simulink model "helicopter_sim"  (R2024b)
settings: Solver=ode4  StartTime=0.0  StopTime=30  FixedStep=ST  RelTol=1e-3
StopFcn:
  | % main rotor flapping restraint
  | if over_flap
  |     warning('MyModel:flapping', '<strong> main rotor blade flapping exceeded limits </strong>');
  | end
  | % tail rotor flapping restraint
  | if over_flap_tr
  |     warning('MyModel:flapping_tr', '<strong> tail rotor blade flapping exceeded limits </strong>');
  | end
  | % main rotor load limit
  | if load_mr
  |     warning('MyModel:load_mr', '<strong> main rotor load limit reached </strong>');
  | end
  | % main rotor power limit
  | if power_mr
  |     warning('MyModel:power_mr', '<strong> transmission maximum power rating reached </strong>');
  | end
  | % main rotor blade stall
  | if stall_mr
  |     warning('MyModel:blade_stall', '<strong> main rotor blade stall </strong>');
  | end
  | clear over_flap over_flap_tr load_mr power_mr stall_mr
values from neighbouring files (symbols this model uses):
  a_0 = [ 0 0 0 ]'*pi/180    [parameters.m]    (also in trim.m = [ flap_ss(1) flap_ss(2) flap_ss(3) ]')
  a_hs = 6    [parameters.m]
  a_vs = 6    [parameters.m]
  AKBETA = 0    [parameters.m]
  AKONE = 0    [parameters.m]
  AKONETR = tan(30*(pi/180))    [parameters.m]
  alpha_stall = 15    [parameters.m]
  AOP = 0    [parameters.m]
  AOPTR = 0    [parameters.m]
  AR_hs = 4.5    [parameters.m]
  AR_vs = 1.8    [parameters.m]
  ASLOPE = 6    [parameters.m]
  ASLOPETR = 6    [parameters.m]
  BLADES = 4    [parameters.m]
  BLADESTR = 3    [parameters.m]
  BLCG = 0    [parameters.m]
  BLHS = 0    [parameters.m]
  BLMR = 0    [parameters.m]
  BLRPF = 0    [parameters.m]
  BLTR = -1.8*Ft_m    (= -0.54864)    [parameters.m]
  BLVS = 0    [parameters.m]
  CD_f = [1.774 0.2043 7]    [parameters.m]
  CD_mr = [0.0107 -0.151 1.72]    [parameters.m]
  CD_tr = [ 0.0107 -0.151 1.72 ]    [parameters.m]
  chi_mr = 1    [parameters.m]
  chi_tr = 1    [parameters.m]
  CHORD = 2*Ft_m    (= 0.6096)    [parameters.m]
  CHORDTR = 1*Ft_m    (= 0.3048)    [parameters.m]
  CL_f = [-0.4279 10.33]    [parameters.m]
  CL_max_hs = 1.2    [parameters.m]
  CL_max_vs = 1.2    [parameters.m]
  CLL_f = [0.0696 6.336]    [parameters.m]
  CM_f = [-4.4961 49.522]    [parameters.m]
  CN_f = [0.0396 -21.699]    [parameters.m]
  CY_f = [-0.0359 -16.987]    [parameters.m]
  D = zeros(9,4)    [linearization.m]
  dyn_viscosity = 17.89e-6    (= 1.789e-05)    [parameters.m]
  e_hs = 0.8    [parameters.m]
  e_vs = 0.8    [parameters.m]
  EPSLN = 0.05    [parameters.m]
  euler0 = [ 0 0 0 ]'*pi/180    [parameters.m]    (also in trim.m = [ euler_trim(1)*abs(max_att) euler_trim(2)*abs(max_att) eule)
  fc = [  100*Kn_mps ... (first row only)    [parameters.m]
  GAMMA = 8.1    [parameters.m]
  GAMMATR = 4    [parameters.m]
  href = 0    [parameters.m]
  i_hs = -3*(pi/180)+a0_hs    (= -0.0523598775598)    [parameters.m]
  i_s = 0    [parameters.m]
  i_vs = 0*(pi/180)+a0_vs    (= -0.0872664625997)    [parameters.m]
  Jbeta = 1/3*m_blade*ROTOR^3*(1-EPSLN)^3    (= 3891.86391298)    [parameters.m]
  k_ind = 1    [parameters.m]
  k_ind_tr = 1    [parameters.m]
  kv_tr = 0.8    [parameters.m]
  Lambda_hs = 13*(pi/180)    (= 0.226892802759)    [parameters.m]
  Lambda_vs = 27*(pi/180)    (= 0.471238898038)    [parameters.m]
  lat_cyc_range = [ -15 15 ]    [parameters.m]
  latref = 39.24744998520548    (= 39.2474499852)    [parameters.m]
  lon_cyc_range = [ -15 15 ]    [parameters.m]
  lonref = 9.050782438199448    (= 9.0507824382)    [parameters.m]
  m = 20000*Lb_Kg    (= 9071.84)    [parameters.m]
  m_blade = 0.372*Slug_Kg/Ft_m    (= 17.8114564173)    [parameters.m]
  max_flap_mr = 20*pi/180    (= 0.349065850399)    [parameters.m]
  max_flap_tr = 20*pi/180    (= 0.349065850399)    [parameters.m]
  max_load = 3*m*9.81    (= 266984.2512)    [parameters.m]
  mode = 0    [linearization.m]    (also in parameters.m; trim.m)
  mr_coll_range = [   0 25 ]    [parameters.m]
  OMEGA = 206.9*(pi/30)    (= 21.6665173343)    [parameters.m]
  omega0 = [ 0 0 0 ]'    [parameters.m]
  OMEGATR = 954.93*(pi/30)    (= 100.000035756)    [parameters.m]
  pilot_trim = [ x(1); x(2); x(3); x(4) ]    [trim.m]
  rated_power = 4170*hp_W    (= 3109569)    [parameters.m]
  ROTOR = 30*Ft_m    (= 9.144)    [parameters.m]
  ROTORTR = 6.5*Ft_m    (= 1.9812)    [parameters.m]
  S_hs = 18*(Ft_m^2)    (= 1.67225472)    [parameters.m]
  S_vs = 33*(Ft_m^2)    (= 3.06580032)    [parameters.m]
  ST = 0.001    [parameters.m]
  STACG = 24.4*Ft_m    (= 7.43712)    [parameters.m]
  STAHS = 57.4*Ft_m    (= 17.49552)    [parameters.m]
  STAMR = 23.9*Ft_m    (= 7.28472)    [parameters.m]
  STARPF = 23.9*Ft_m    (= 7.28472)    [parameters.m]
  STATR = 61.4*Ft_m    (= 18.71472)    [parameters.m]
  STAVS = 59.4*Ft_m    (= 18.10512)    [parameters.m]
  THETT = -10*(pi/180)    (= -0.174532925199)    [parameters.m]
  THETTTR = -5*(pi/180)    (= -0.0872664625997)    [parameters.m]
  tr_coll_range = [   0 20 ]    [parameters.m]
  Ttrb = [ 1 0 0; 0 0 1; 0 -1 0]    [parameters.m]
  V0 = eul2rotm(euler0','XYZ')'*[ fc(1) fc(2) fc(3) ]'    [parameters.m]    (also in trim.m)
  wind_rate = [ 0 0 0 ]'    [parameters.m]
  wind_velocity_e = [ 0 0 0 ]'    [parameters.m]
  WLCG = 9.2*Ft_m    (= 2.80416)    [parameters.m]
  WLHS = 7.7*Ft_m    (= 2.34696)    [parameters.m]
  WLMR = 16.7*Ft_m    (= 5.09016)    [parameters.m]
  WLRPF = 12.2*Ft_m    (= 3.71856)    [parameters.m]
  WLTR = 15.2*Ft_m    (= 4.63296)    [parameters.m]
  WLVS = 12.2*Ft_m    (= 3.71856)    [parameters.m]
  Xe_0 = [ 16404 0 -1000 ]'*Ft_m    [parameters.m]
undefined symbols (not defined in the file or in its folder): Earth, rad, s, WGS84
libraries: simulink x4, aerolibanimutils x2, aerolibsim3d x2, sim3dlib x1, aerolibconvert2 x1, shared6dof x1, aerolibtransform2 x1, aerolibatmos2 x1
(part 3 of 3)

== matlab function helicopter_sim/HELICOPTER MODEL/HELICOPTER FORCES AND MOMENTS/MAIN ROTOR/AERODYNAMIC AND INERTIAL FORCES AND MOMENTS ==
  data: chi input; i_s input; m_blade input; Jbeta input; GAMMA input; EPSLN input; AKBETA input; g input; BLADES input; Mrotor output; ASLOPE input; AKONE input; CHORD input; CD input; ROTOR input; A1s input; B1s input; a0 input; a1 input; b1 input; a0dot input; a1dot input; b1dot input; a0ddot input; a1ddot input; b1ddot input; Theta0 input; THETT input; dyn_viscosity input; k_ind input; STACG input; BLCG input; WLCG input; STAH input; BLH input; WLH input; rho input; TAS input; omega_TAS input; Frotor output; omega input; OMEGA input; lambda_i output; lambda output; T output; Q output; alpha_loc output
function [Mrotor,Frotor,lambda_i,lambda,T,Q,alpha_loc]  = fcn(chi,i_s,m_blade,Jbeta,GAMMA,EPSLN,AKBETA,g,BLADES,ASLOPE,AKONE,CHORD,CD,ROTOR,A1s,B1s,...
                                                                    a0,a1,b1,a0dot,a1dot,b1dot,a0ddot,a1ddot,b1ddot,Theta0,THETT,dyn_viscosity,k_ind,...
                                                                    STACG,BLCG,WLCG,STAH,BLH,WLH,rho,TAS,omega_TAS,omega,OMEGA)

%% preliminary calculations
A = pi*ROTOR^2; % area of rotor disc 
sigma = BLADES*CHORD/(pi*ROTOR); % solidity of rotor 
lever_arm_H = [STACG-STAH BLH-BLCG WLCG-WLH]'; % vector from cg to rotor hub
TAS_H = [1 chi 1]'.*(TAS + cross(omega_TAS,lever_arm_H)); % wind speed at rotor
% rotation of airspeed from body to hub-body frame:
uH = TAS_H(1)*cos(i_s)-TAS_H(3)*sin(i_s);
vH = TAS_H(2);
wH = TAS_H(1)*sin(i_s)+TAS_H(3)*cos(i_s);
beta_w = atan2(vH,uH); % sideslip angle 
Mu = sqrt(uH^2+vH^2)/(OMEGA*ROTOR); % advance ratio
p = omega(1); % roll rate
q = omega(2); % pitch rate
r = omega(3); % yaw rate
% rotation of body angular rates from body to hub-body frame:
pH = chi*(p*cos(i_s)+r*sin(i_s));
qH = q;
% rotation of body angular rates from hub-body to hub-wind frame:
pW = pH*cos(beta_w)+qH*sin(beta_w);
qW = -pH*sin(beta_w)+qH*cos(beta_w);
% rotation of feathering angles from hub-body to hub-wind frame:
A1c = A1s*cos(beta_w)-B1s*sin(beta_w);
B1c = A1s*sin(beta_w)+B1s*cos(beta_w);
Mbeta = g*1/2*m_blade*ROTOR^2*(1-EPSLN)^2; % weight moment of the blade around flap hinge (small flapping angle beta and level attitude) 
                                           % (distance from blade c.g. to flap hinge)*(blade weight) [N*m]
                                           % small contribution to the coning angle, can be neglected

%% thrust and inflow calculation

lambda = fzero(@(x) x-wH/(OMEGA*ROTOR)+0.5*(0.5*BLADES*rho*ASLOPE*CHORD*ROTOR*(OMEGA*ROTOR)^2*(1/2*(1-EPSLN^2)*x+Theta0*(1/3+Mu^2/2*(1-EPSLN))+THETT*(1/4+Mu^2/4*(1-EPSLN^2))+...
                    -Mu/2*(1-EPSLN^2)*(B1c-AKONE*b1)-a0*(1/3+Mu^2/2*(1-EPSLN))*AKONE+a1*(Mu/2*EPSLN*(1-EPSLN))-a0dot/OMEGA*(1/3-EPSLN/2)+b1dot/OMEGA*(Mu/4*(1-EPSLN)^2)+...
                    +Mu/4*(1-EPSLN^2)*pW/OMEGA)-BLADES*Mbeta/g*a0ddot)/(rho*A*(OMEGA*ROTOR)^2)/sqrt(Mu^2+x^2), -0.1);
vi = wH-lambda*OMEGA*ROTOR;
lambda_i = -vi/OMEGA/ROTOR;
T =  0.5*BLADES*rho*ASLOPE*CHORD*ROTOR*(OMEGA*ROTOR)^2*(1/2*(1-EPSLN^2)*lambda+Theta0*(1/3+Mu^2/2*(1-EPSLN))+THETT*(1/4+Mu^2/4*(1-EPSLN^2))+...
     -Mu/2*(1-EPSLN^2)*(B1c-AKONE*b1)-a0*(1/3+Mu^2/2*(1-EPSLN))*AKONE+a1*(Mu/2*EPSLN*(1-EPSLN))-a0dot/OMEGA*(1/3-EPSLN/2)+b1dot/OMEGA*(Mu/4*(1-EPSLN)^2)+...
     +Mu/4*(1-EPSLN^2)*pW/OMEGA)-BLADES*Mbeta/g*a0ddot;
CT = T/(rho*A*(OMEGA*ROTOR)^2);
V = sqrt(vi^2+(OMEGA*ROTOR)^2);
Re = rho*CHORD*V/dyn_viscosity; % Reynolds number based on tip speed and rotor chord
alpha_mean = 6*CT/ASLOPE/sigma;
delta = CD(1)+CD(2)*alpha_mean+CD(3)*alpha_mean^2;

%% forces and moments in the hub-wind frame

H_w = BLADES/2*rho*ASLOPE*CHORD*ROTOR*(OMEGA*ROTOR)^2*(delta*Mu/(2*ASLOPE)*(1-EPSLN^2)-1/4*(Theta0-AKONE*a0)*(2*lambda*Mu*(1-EPSLN)+ ...
      -Mu*(1-EPSLN)^2*a0dot/OMEGA-(EPSLN-2/3)*(b1dot/OMEGA-a1)-2/3*a1+2/3*pW/OMEGA)-THETT/4*(Mu*lambda*(1-EPSLN^2)+a0dot/OMEGA*Mu*(EPSLN-2/3)+...
      -2*(EPSLN/3-1/4)*(b1dot/OMEGA-a1)-a1/2+1/2*pW/OMEGA)+1/4*(A1c-AKONE*a1)*(-b1*Mu/4*(1-EPSLN^2)+1/4*Mu*(1-EPSLN)^2*(a1dot/OMEGA+b1)+2/3*a0+...
      +Mu/4*(1-EPSLN^2)*qW/OMEGA)+1/4*(B1c-AKONE*b1)*(3/4*Mu*(1-EPSLN)^2*(b1dot/OMEGA-a1)+(1-EPSLN^2)*(lambda-a1*Mu/4)+(EPSLN-2/3)*a0dot/OMEGA+...
      +3*Mu/4*(1-EPSLN^2)*pW/OMEGA)+1/4*(EPSLN*(1-EPSLN)*(b1dot/OMEGA-a1)*4*lambda-(1-EPSLN^2)*(2*lambda*(b1dot/OMEGA-a1)-a1*lambda)+...
      -(2/3-EPSLN)*(a1*a0dot/OMEGA+a0*(a1dot/OMEGA+b1))-2*a0/3*qW/OMEGA-(2*(1-EPSLN^2)*lambda-4*(1/3-EPSLN/2)*a0dot/OMEGA)*pW/OMEGA+...
      +4*a0dot/OMEGA*(b1dot/OMEGA-a1)*(1/3-EPSLN+EPSLN^2))+Mu/4*(EPSLN*(1-EPSLN)*(a1*(b1dot/OMEGA-a1)+b1*(a1dot/OMEGA+b1))+...
      +1/4*(1-EPSLN)^2*(b1*(a1dot/OMEGA+b1)+a1*(b1dot/OMEGA-a1))-1/2*(1-EPSLN^2)*(a1*(b1dot/OMEGA-a1)+b1*(a1dot/OMEGA+b1)-2*a0^2-b1^2/2-3/2*a1^2)+...
      -a1/4*(1-EPSLN^2)*pW/OMEGA-b1/4*(1-EPSLN^2)*qW/OMEGA));

Y_w = BLADES/2*rho*ASLOPE*CHORD*ROTOR*(OMEGA*ROTOR)^2*(-1/4*(Theta0-AKONE*a0)*(((EPSLN-2/3)*(a1dot/OMEGA+b1)-2/3*b1)+3*a0*(1-EPSLN^2)*Mu+ ...
      -2*b1*(1-EPSLN)*Mu^2-2/3*qW/OMEGA)-THETT/4*(((2/3*EPSLN-1/2)*(a1dot/OMEGA+b1)-b1/2)+2*a0*Mu-b1*(1-EPSLN^2)*Mu^2+ ...
      -1/2*qW/OMEGA)-1/4*(A1c-AKONE*a1)*(((EPSLN-2/3)*a0dot/OMEGA+lambda*(1-EPSLN^2))+Mu*(5/4*a1*(1-EPSLN^2)+1/4*(1-EPSLN)^2*(b1dot/OMEGA-a1))+...
      +Mu/4*(1-EPSLN^2)*pW/OMEGA)-1/4*(B1c-AKONE*b1)*(-2/3*a0+Mu*(7/4*b1*(1-EPSLN^2)+1/4*(1-EPSLN)^2*(a1dot/OMEGA+b1)+...
      +1/4*qW/OMEGA)-Mu^2*(2*a0*(1-EPSLN)))-1/4*(4*(1/3-EPSLN+EPSLN^2)*a0dot/OMEGA*(a1dot/OMEGA+b1)-2*lambda*(1-EPSLN)^2*(a1dot/OMEGA+b1)+...
      +2/3*a0*pW/OMEGA+2*a0*(1/3-EPSLN/2)*(b1dot/OMEGA-a1)-2*b1*(lambda/2*(1-EPSLN^2)-a0dot/OMEGA*(1/3-EPSLN/2))+(4*(1/3-EPSLN/2)*a0dot/OMEGA+...
      -2*(1-EPSLN^2)*lambda)*qW/OMEGA)-Mu/4*(6*a0*lambda*(1-EPSLN)-a1*b1/2*(1-EPSLN^2)-3*(1-EPSLN)^2*a0*a0dot/OMEGA-7/4*(1-EPSLN)^2*a1*(a1dot/OMEGA+b1)+...
      -5/4*b1*(1-EPSLN^2)*pW/OMEGA-7/4*a1*(1-EPSLN^2)*qW/OMEGA-5/4*(1-EPSLN)^2*b1*(b1dot/OMEGA-a1))-Mu^2*(a0*a1*(1-EPSLN)));

M_w = BLADES/2*(AKBETA*a1-EPSLN*ROTOR*Mbeta/g*(a1ddot+2*b1dot*OMEGA-a1*OMEGA^2))-BLADES/2*Jbeta*OMEGA^2*GAMMA*EPSLN*(-(1/6+Mu^2/8*(1-EPSLN))*(A1c-AKONE*a1)+...
      -Mu/4*(1-EPSLN^2)*a0+Mu^2/8*(1-EPSLN)*b1+(1/6-EPSLN/4)*(a1dot/OMEGA+b1)+1/6*qW/OMEGA);

L_w = BLADES/2*(AKBETA*b1-EPSLN*ROTOR*Mbeta/g*(b1ddot-2*a1dot*OMEGA-b1*OMEGA^2))-BLADES/2*Jbeta*OMEGA^2*GAMMA*EPSLN*(Mu/2*(1-EPSLN^2)*(Theta0-AKONE*a0)+...
      -(1/6+3/8*Mu^2*(1-EPSLN))*(B1c-AKONE*b1)+Mu/3*THETT+Mu/2*(1-EPSLN)*lambda+Mu^2/8*(1-EPSLN)*a1-Mu/4*(1-EPSLN)^2*a0dot/OMEGA+(1/6-EPSLN/4)*(b1dot/OMEGA-a1)+1/6*pW/OMEGA);

Q = k_ind*BLADES/2*rho*ASLOPE*CHORD*ROTOR^2*(OMEGA*ROTOR)^2*(delta/k_ind/(4*ASLOPE)*(1+(1-EPSLN^2)*Mu^2)-(Theta0-AKONE*a0)*(lambda/3+(EPSLN/3-1/4)*a0dot/OMEGA+...
    +Mu/6*b1dot/OMEGA-Mu*EPSLN/4*(b1dot/OMEGA-a1)+Mu/6*pW/OMEGA)+(A1c-AKONE*a1)*((1/8-EPSLN/6)*(a1dot/OMEGA+b1)-Mu/6*a0+b1/16*(1-EPSLN^2)*Mu^2+1/8*qW/OMEGA)+...
    +(B1c-AKONE*b1)*((1/8-EPSLN/6)*(b1dot/OMEGA-a1)+(EPSLN/4-1/6)*Mu*a0dot/OMEGA+1/2*(1-EPSLN^2)*(Mu*lambda/2+a1/8*Mu^2)+1/8*pW/OMEGA)-THETT*(lambda/4+...
    +(EPSLN/4-1/5)*a0dot/OMEGA+Mu/8*b1dot/OMEGA-EPSLN*Mu/6*(b1dot/OMEGA-a1))-1/2*(1-EPSLN^2)*(lambda^2+lambda*Mu*a1+2*lambda*EPSLN*a0dot/OMEGA+...
    +Mu*EPSLN*(a1*a0dot/OMEGA+a0*(a1dot/OMEGA+b1))+Mu^2*(a0^2/2+3/8*a1^2+1/8*b1^2))+Mu/3*(a1*a0dot/OMEGA+a0*(a1dot/OMEGA+b1))+2/3*lambda*a0dot/OMEGA+...
    -(-Mu/3*a0+(1/4-EPSLN/3)*(a1dot/OMEGA+b1))*qW/OMEGA-(1/4-EPSLN/3)*(b1/OMEGA-a1)*pW/OMEGA-1/8*(qW/OMEGA)^2-1/8*(pW/OMEGA)^2-(1/4-2/3*EPSLN+EPSLN^2/2)*((a0dot/OMEGA)^2+...
    +1/2*((a1dot/OMEGA+b1)^2+(b1dot/OMEGA-a1)^2)));


%% back rotation from hub_wind frame to hub-frame

H_H = H_w*cos(beta_w)+Y_w*sin(beta_w);
Y_H = -H_w*sin(beta_w)+Y_w*cos(beta_w);
L_H = L_w*cos(beta_w)-M_w*sin(beta_w);
M_H = L_w*sin(beta_w)+M_w*cos(beta_w);

%% back rotation from hub-frame to body-frame

X = T*sin(i_s)-H_H*cos(i_s);
Y = chi*Y_H;
Z = -T*cos(i_s)-H_H*sin(i_s);
Frotor = [X Y Z]';

L_MR = L_H*cos(i_s)-Q*sin(i_s);
M_MR = M_H;
N_MR = Q*cos(i_s)+L_H*sin(i_s);
Mrotor = [chi*L_MR M_MR chi*N_MR]'+cross(lever_arm_H,Frotor);

%% blade element angle of attack in hub-wind axis
% angle of attack of tip path plane (positive nose up):
if sqrt(uH^2+vH^2+wH^2) == 0
    alpha_tpp = 0;
else
    alpha_tpp = a1+asin(wH/sqrt(uH^2+vH^2+wH^2)); 
end

psi    = linspace(0,360,10).*pi/180; % azimuth, positive ccw, 90deg at advancing side
radius = linspace(0.2*ROTOR,ROTOR,5); % radial stations
[psi,radius] = meshgrid(psi,radius); % transform to meshgrid coordinates
% local blade angle of attack [deg]:
alpha_loc = (1./((radius./ROTOR)+Mu.*sin(psi))).*...
            ((radius./ROTOR).*(Theta0+THETT.*(radius./ROTOR)-(A1c-b1).*cos(psi)-(B1c+a1).*sin(psi))+...
            lambda_i.*(1+(radius./ROTOR).*cos(psi))+Mu.*...
            (alpha_tpp+(Theta0+THETT.*(radius./ROTOR))...
            .*sin(psi)-a0.*cos(psi)-(A1c-b1).*sin(psi).*cos(psi)...
            -(B1c+a1).*(sin(psi)).^2)).*180/pi;
